simulink model "TC_Uno_MRC_MIT_Rule"  (R2018b)
settings: Solver=ode2  StartTime=0.0  StopTime=inf  FixedStep=1e-3  RelTol=1e-3  EnableMultiTasking=on
libraries: arduinolib x2
settings Model: SimulationMode=external  ExtModeTrigDuration=2  Creator=user  LastModifiedBy=auralius
settings OptimizationCC: EnhancedBackFolding=on  PassReuseOutputArgsAs=Individual arguments  MaxStackSize=64  OptimizeBlockOrder=speed  DifferentSizesBufferReuse=on  OptimizationCustomize=off
settings DebuggingCC: ParameterTunabilityLossMsg=error  LibraryContextMissingDiagnostic=none
settings HardwareCC: ProdBitPerInt=16  ProdBitPerPointer=16  ProdBitPerSizeT=16  ProdBitPerPtrDiffT=16  ProdLargestAtomicFloat=None  ProdWordSize=8  ProdHWDeviceType=Atmel->AVR
settings SFSimCC: SimCustomTerminator=analogWrite(9, 0);  SimUseLocalCustomCode=off  MATLABDynamicMemAlloc=off
settings RTWCC: SystemTargetFile=ert.tlc  HardwareBoard=Arduino Mega 2560  TemplateMakefile=ert_default_tmf  GenerateReport=on  RTWUseLocalCustomCode=off  Toolchain=Arduino AVR  BuildConfiguration=Faster Runs  IncludeHyperlinkInReport=on  LaunchReport=on  GenerateTraceInfo=on  GenerateTraceReport=on  GenerateTraceReportSl=on  GenerateTraceReportSf=on  GenerateTraceReportEml=on
settings CodeAppCC: ForceParamTrailComments=on  IgnoreCustomStorageClasses=off  OperatorAnnotations=on  SimulinkDataObjDesc=on  SFDataObjDesc=on  InsertBlockDesc=on
settings ERTTargetCC: SupportContinuousTime=on  SupportVariableSizeSignals=on  ExtMode=on  ExtModeMexArgs='127.0.0.1' 0 17725

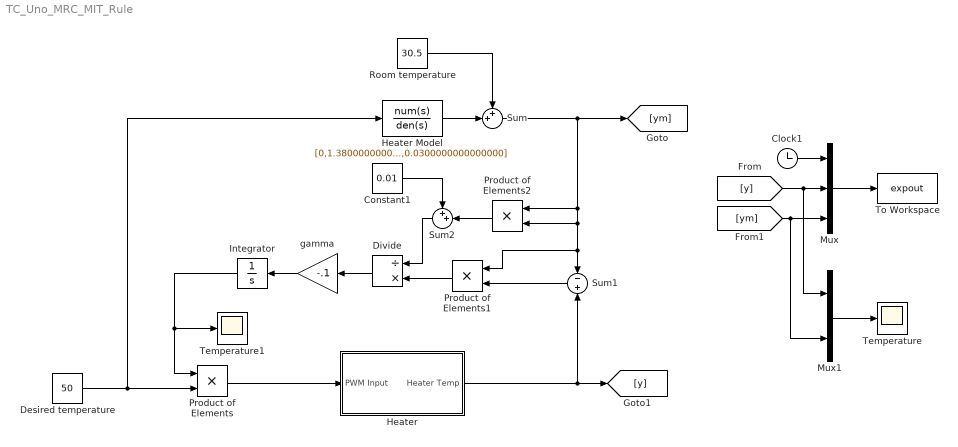
== system TC_Uno_MRC_MIT_Rule ==
  Clock1 : Clock
  Constant1 : Constant  Value=0.01
  Desired temperature : Constant  Value=50
  Divide : Product  Inputs=/*
  Heater : Subsystem
  Heater Model : TransferFcn  Numerator=[0,1.38000000000000,-0.414000000000000,0.0414000000000000]  Denominator=[212.200000000000,64.6600000000000,6.66600000000000,0.0300000000000000]
  Integrator : Integrator
  Mux : Mux  Inputs=3
  Mux1 : Mux  Inputs=2
  Product of Elements : Product
  Product of Elements1 : Product
  Product of Elements2 : Product
  Room temperature : Constant  Value=30.5
  Sum : Sum  Inputs=++|
  Sum1 : Sum  Inputs=-|+
  Sum2 : Sum  Inputs=++|
  Temperature : Scope
  Temperature1 : Scope
  To Workspace : ToWorkspace  VariableName=expout  SampleTime=-1
  gamma : Gain  Gain=-.1
  wires:
  Desired temperature/1 -> Heater Model/1, Product of Elements/2
  Heater Model/1 -> Sum/2
  Integrator/1 -> Temperature1/1, Product of Elements/1
  gamma/1 -> Integrator/1
  Heater/1(Heater Temp) -> [y], Sum1/2
  Sum1/1 -> Product of Elements1/2
  Product of Elements/1 -> Heater/1(PWM Input)
  Room temperature/1 -> Sum/1
  Sum/1 -> Product of Elements2/1, Product of Elements2/2, Sum1/1, Product of Elements1/1, [ym]
  Mux/1 -> To Workspace/1
  Clock1/1 -> Mux/1
  [y] -> Mux1/1, Mux/2
  [ym] -> Mux1/2, Mux/3
  Mux1/1 -> Temperature/1
  Product of Elements2/1 -> Sum2/2
  Constant1/1 -> Sum2/1
  Sum2/1 -> Divide/1
  Product of Elements1/1 -> Divide/2
  Divide/1 -> gamma/1

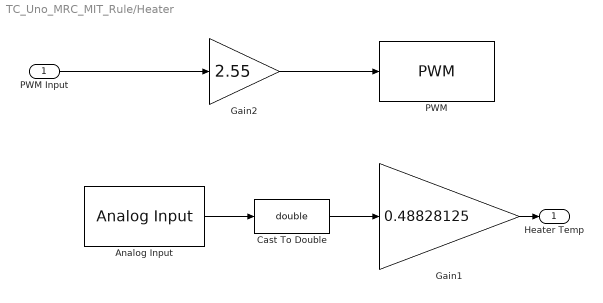
== system TC_Uno_MRC_MIT_Rule/Heater ==
  PWM Input : Inport
  Analog Input : arduinolib/Analog Input  pinNumber=0  ReadResultsOnly=off  ConversionTriggerSource=Software  ExternalTriggerType=uint32(0)  OutputDataType=uint16  EnableConversionCompleteNotify=off  EnableOuputStatus=off  SampleTime=-1  blockPlatform=arduino
  Cast To Double : DataTypeConversion  OutDataTypeStr=double
  Gain1 : Gain  Gain=0.48828125
  Gain2 : Gain  Gain=2.55
  PWM : arduinolib/PWM  pinNumber=9  EnableInputFrequency=off  InitialFrequency=2000  InitialDutyCycle=0  NotificationType=None  blockPlatform=arduino
  Heater Temp : Outport
  wires:
  Analog Input/1 -> Cast To Double/1
  Cast To Double/1 -> Gain1/1
  Gain1/1 -> Heater Temp/1
  PWM Input/1 -> Gain2/1
  Gain2/1 -> PWM/1
